simulink model "nczallcode"  (R2024a)
settings: Solver=FixedStepAuto  StartTime=0.0  StopTime=600  FixedStep=1  RelTol=1e-3
model workspace (MAT data in the model file):
  avg_loc = []
  first_column1 = []
  first_column6 = []
  locs = []
  maxValue = []
  newMaxIndex = []
  peaks = []
  stdNum = []
settings Model: Creator=LiGuoQing  LastModifiedBy=PC
settings OptimizationCC: DefaultParameterBehavior=Inlined  EnhancedBackFolding=on  PassReuseOutputArgsAs=Individual arguments  ZeroExternalMemoryAtStartup=off  ZeroInternalMemoryAtStartup=off  OptimizeBlockOrder=speed  DifferentSizesBufferReuse=on  OptimizationCustomize=off  EfficientTunableParamExpr=on
settings DebuggingCC: ParameterTunabilityLossMsg=error  UnconnectedInputMsg=warning  UnconnectedOutputMsg=warning  UnconnectedLineMsg=warning
settings HardwareCC: ProdBitPerPointer=32  ProdBitPerSizeT=32  ProdBitPerPtrDiffT=32  ProdLargestAtomicInteger=Long  ProdLargestAtomicFloat=Double  ProdWordSize=32  ProdHWDeviceType=NXP->Cortex-M4
settings ModelReferenceCC: EnableRefExpFcnMdlSchedulingChecks=on
settings SFSimCC: MATLABDynamicMemAlloc=off
settings RTWCC: Description=Embedded Coder  SystemTargetFile=ert.tlc  GenCodeOnly=on  TemplateMakefile=ert_default_tmf  GenerateReport=on  Toolchain=Microsoft Visual C++ 2019 v16.0 | nmake (64-bit Windows)  LaunchReport=on  GenerateWebview=on  GenerateCodeMetricsReport=on  GPUComputeCapability=3.5  DLArmComputeVersion=19.05
settings CodeAppCC: ForceParamTrailComments=on  IgnoreCustomStorageClasses=off  OperatorAnnotations=on  SimulinkDataObjDesc=on  SFDataObjDesc=on  InsertBlockDesc=on
settings ERTTargetCC: TargetLangStandard=C99 (ISO)  GenerateSampleERTMain=on  SupportContinuousTime=on  SupportVariableSizeSignals=on  InlinedParameterPlacement=NonHierarchical  RootIOFormat=Structure reference  ERTCustomFileTemplate=example_file_process.tlc

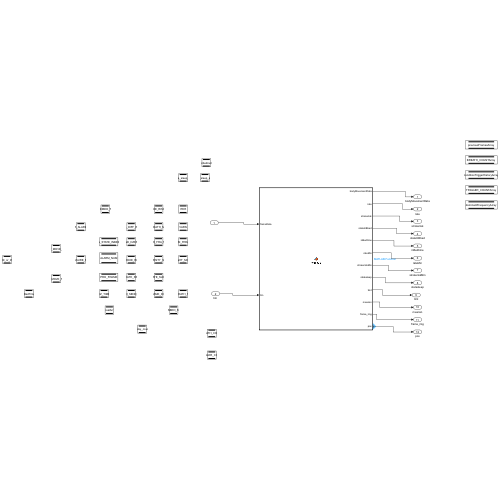
[thumbnail: Simulink's stored preview of the top-level diagram]
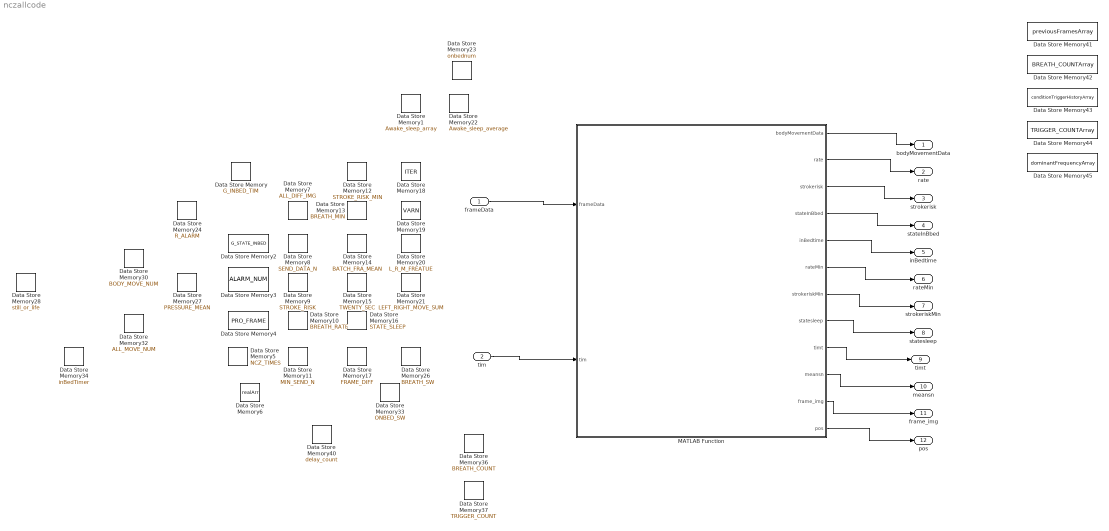
== system nczallcode ==
  frameData : Inport  OutDataTypeStr=single  PortDimensions=160
  "tim " : Inport  Port=2  OutDataTypeStr=single
  Data Store Memory : DataStoreMemory  DataStoreName=G_INBED_TIM  ReadBeforeWriteMsg=warning  WriteAfterWriteMsg=warning  WriteAfterReadMsg=warning  ShowAdditionalParam=off  OutDataTypeStr=single
  Data Store Memory1 : DataStoreMemory  DataStoreName=Awake_sleep_array  ReadBeforeWriteMsg=warning  WriteAfterWriteMsg=warning  WriteAfterReadMsg=warning  InitialValue=ones(1, 300)  ShowAdditionalParam=off  OutDataTypeStr=single
  Data Store Memory10 : DataStoreMemory  DataStoreName=BREATH_RATE  ReadBeforeWriteMsg=warning  WriteAfterWriteMsg=warning  WriteAfterReadMsg=warning  ShowAdditionalParam=off  OutDataTypeStr=single
  Data Store Memory11 : DataStoreMemory  DataStoreName=MIN_SEND_N  ReadBeforeWriteMsg=warning  WriteAfterWriteMsg=warning  WriteAfterReadMsg=warning  ShowAdditionalParam=off  OutDataTypeStr=single
  Data Store Memory12 : DataStoreMemory  DataStoreName=STROKE_RISK_MIN  ReadBeforeWriteMsg=warning  WriteAfterWriteMsg=warning  WriteAfterReadMsg=warning  ShowAdditionalParam=off  OutDataTypeStr=single
  Data Store Memory13 : DataStoreMemory  DataStoreName=BREATH_MIN  ReadBeforeWriteMsg=warning  WriteAfterWriteMsg=warning  WriteAfterReadMsg=warning  ShowAdditionalParam=off  OutDataTypeStr=single
  Data Store Memory14 : DataStoreMemory  DataStoreName=BATCH_FRA_MEAN  ReadBeforeWriteMsg=warning  WriteAfterWriteMsg=warning  WriteAfterReadMsg=warning  InitialValue=[0,0,0,0,0,0,0,0,0,0,0,0,0,0,0,0,0,0,0,0,0,0,0,0,0,0,0,0,0,0,0,0,0,0,0,0,0,0,0,0,0,0,0,0,0,0,0,0,0,0,0,0,0,0,0,0,0,0,0,0,0,0,0,0,0,0,0,0,0,0,0,0,0,0,0,0,0,0,0,0,0,0,0,0,0,0,0,0,0,0,0,0,0,0,0,0,0,0,0,0,0,0,0,0,0,0,0,0,0,0,0,0,0,0,0,0,0,0,0,0,0,0,0,0,0,0,0,0,0,0,0,0,0,0,0,0,0,0,0,0,0,0,0,0,0,0,0,0,0,0,0,0,0,0,0,0,0,0,0,0,0,0,0,0,0,0,0,0,0,0,0,0,0,0,0,0,0,0,0,0,0,0,0,0,0,0,0,0,0,0,0,0,0,0,0,0,0,0,0,0,0,0,0,0,0,0,0,0,0,0,0,0,0,0,0,0,0,0,0,0,0,0,0,0,0,0,0,0,0,0,0,0,0,0,0,0,0,0,0,0,0,0,0,0,0,0,0,0,0,0,0,0,0,0,0,0,0,0,0,0,0,0,0,0,0,0,0,0,0,0,0,0,0,0,0,0,0,0,0,0,0,0,0,0,0,0,0,0,0,0,0,0,0,0,0,0,0,0,0,0,0,0,0,0,0,0,0,0,0,0,0,0,0,0,0,0,0,0,0,0,0,0,0,0,0,0,0,0,0,0,0,0,0,0,0,0,0,0,0,0,0,0,0,0,0,0,0,0,0,0,0,0,0,0,0,0,0,0,0,0,0,0,0,0,0,0,0,0,0,0,0,0,0,0,0,0,0,0,0,0,0,0,0,0,0,0,0,0,0,0,0,0,0,0,0,0,0,0,0,0,0,0,0,0,0,0,0,0,0,0,0,0,0,0,0,0,0,0,0,0,0,0,0,0,0,0,0,0,0,0,0,0,0,0,0,0,0,0,0,0,0,0,0,0,0,0,0,0,0,0,0,0,0,0,0,0,0,0,0,0,0,0,0,0,0,0,0,0,0,0,0,0,0,0,0,0,0,0,0,0,0,0,0,0,0,0,0,0,0,0,0,0,0,0,0,0,0,0,0,0,0,0,0,0,0,0,0,0,0,0,0,0,0,0,0,0,0,0,0,0,0,0,0,0,0,0,0,0,0,0,0,0,0,0,0,0,0,0,0,0,0,0,0,0,0,0,0,0,0,0,0,0,0,0,0,0,0,0,0,0,0,0,0,0,0,0,0,0,0,0,0,0,0,0,0,0,0,0,0,0,0,0,0,0,0,0,0,0,0,0,0,0,0,0,0,0,0,0,0,0,0,0,0,0,0,0,0,0,0,0,0,0,0,0,0,0,0,0,0,0,0,0,0,0,0,0,0,0,0,0,0,0,0,0,0,0,0,0,0,0,0,0,0,0,0,0,0,0,0,0,0,0,0,0,0,0,0,0,0,0,0,0,0,0,0,0,0,0,0,0,0,0,0,0,0,0,0,0,0,0,0,0,0,0,0,0,0,0,0,0,0,0,0,0,0,0,0,0,0,0,0,0,0,0,0,0,0,0,0,0,0,0,0,0,0,0,0,0,0,0]  ShowAdditionalParam=off  OutDataTypeStr=single
  Data Store Memory15 : DataStoreMemory  DataStoreName=TWENTY_SEC  ReadBeforeWriteMsg=warning  WriteAfterWriteMsg=warning  WriteAfterReadMsg=warning  ShowAdditionalParam=off  OutDataTypeStr=single
  Data Store Memory16 : DataStoreMemory  DataStoreName=STATE_SLEEP  ReadBeforeWriteMsg=warning  WriteAfterWriteMsg=warning  WriteAfterReadMsg=warning  InitialValue=[0,0,0,0,0,0,0,0,0,0,0,0,0,0,0,0,0,0,0,0,0,0,0,0,0,0,0,0,0,0,0,0,0,0,0,0,0,0,0,0,0,0,0,0,0,0,0,0]  ShowAdditionalParam=off  OutDataTypeStr=single
  Data Store Memory17 : DataStoreMemory  DataStoreName=FRAME_DIFF  ReadBeforeWriteMsg=warning  WriteAfterWriteMsg=warning  WriteAfterReadMsg=warning  InitialValue=[0,0,0,0,0,0,0,0,0,0,0,0,0,0,0,0]  ShowAdditionalParam=off  OutDataTypeStr=single
  Data Store Memory18 : DataStoreMemory  DataStoreName=ITER  ReadBeforeWriteMsg=warning  WriteAfterWriteMsg=warning  WriteAfterReadMsg=warning  ShowAdditionalParam=off  OutDataTypeStr=single
  Data Store Memory19 : DataStoreMemory  DataStoreName=VARN  ReadBeforeWriteMsg=warning  WriteAfterWriteMsg=warning  WriteAfterReadMsg=warning  InitialValue=1  ShowAdditionalParam=off  OutDataTypeStr=single
  Data Store Memory2 : DataStoreMemory  DataStoreName=G_STATE_INBED  ReadBeforeWriteMsg=warning  WriteAfterWriteMsg=warning  WriteAfterReadMsg=warning  ShowAdditionalParam=off  OutDataTypeStr=single
  Data Store Memory20 : DataStoreMemory  DataStoreName=L_R_M_FREATUE  ReadBeforeWriteMsg=warning  WriteAfterWriteMsg=warning  WriteAfterReadMsg=warning  InitialValue=[0,0,0,0,0,0,0,0,0,0,0,0,0,0,0,0,0,0,0,0,0,0,0,0,0,0,0,0,0,0,0,0,0,0,0,0,0,0,0,0,0,0,0,0,0,0,0,0,0,0,0,0,0,0,0,0,0,0,0,0,0,0,0,0,0,0,0,0,0,0,0,0,0,0,0,0,0,0,0,0,0,0,0,0,0,0,0,0,0,0,0,0,0,0,0,0,0,0,0,0,0,0,0,0,0,0,0,0,0,0,0,0,0,0,0,0,0,0,0,0,0,0,0,0,0,0,0,0,0,0,0,0,0,0,0,0,0,0,0,0,0,0,0,0,0,0,0,0,0,0,0,0,0,0,0,0,0,0,0,0,0,0,0,0,0,0,0,0,0,0,0,0,0,0,0,0,0,0,0,0]  ShowAdditionalParam=off  OutDataTypeStr=single
  Data Store Memory21 : DataStoreMemory  DataStoreName=LEFT_RIGHT_MOVE_SUM  ReadBeforeWriteMsg=warning  WriteAfterWriteMsg=warning  WriteAfterReadMsg=warning  InitialValue=[0,0,0,0]  ShowAdditionalParam=off  OutDataTypeStr=single
  Data Store Memory22 : DataStoreMemory  DataStoreName=Awake_sleep_average  ReadBeforeWriteMsg=warning  WriteAfterWriteMsg=warning  WriteAfterReadMsg=warning  InitialValue=zeros(1,48)  ShowAdditionalParam=off  OutDataTypeStr=double
  Data Store Memory23 : DataStoreMemory  DataStoreName=onbednum  ReadBeforeWriteMsg=warning  WriteAfterWriteMsg=warning  WriteAfterReadMsg=warning  ShowAdditionalParam=off  OutDataTypeStr=double
  Data Store Memory24 : DataStoreMemory  DataStoreName=R_ALARM  ReadBeforeWriteMsg=warning  WriteAfterWriteMsg=warning  WriteAfterReadMsg=warning  InitialValue=[0,0,0,0,0,0,0,0,0,0,0,0,0,0,0,0,0,0,0,0,0,0,0,0,0,0,0,0,0,0,0,0,0,0,0,0,0,0,0,0,0,0,0,0,0,0,0,0,0,0,0,0,0,0,0,0,0,0,0,0,0,0,0,0,0,0,0,0,0,0,0,0,0,0,0,0,0,0,0,0,0,0,0,0,0,0,0,0,0,0,0,0,0,0,0,0,0,0,0,0,0,0,0,0,0,0,0,0,0,0,0,0,0,0,0,0,0,0,0,0,0,0,0,0,0,0,0,0,0,0,0,0,0,0,0,0,0,0,0,0,0,0,0,0,0,0,0,0,0,0,0,0,0,0,0,0,0,0,0,0,0,0,0,0,0,0,0,0,0,0,0,0,0,0,0,0,0,0,0,0]  ShowAdditionalParam=off  OutDataTypeStr=single
  Data Store Memory26 : DataStoreMemory  DataStoreName=BREATH_SW  ReadBeforeWriteMsg=warning  WriteAfterWriteMsg=warning  WriteAfterReadMsg=warning  ShowAdditionalParam=off  OutDataTypeStr=single
  Data Store Memory27 : DataStoreMemory  DataStoreName=PRESSURE_MEAN  ReadBeforeWriteMsg=warning  WriteAfterWriteMsg=warning  WriteAfterReadMsg=warning  ShowAdditionalParam=off  OutDataTypeStr=single
  Data Store Memory28 : DataStoreMemory  DataStoreName=still_or_life  ReadBeforeWriteMsg=warning  WriteAfterWriteMsg=warning  WriteAfterReadMsg=warning  ShowAdditionalParam=off  OutDataTypeStr=single
  Data Store Memory3 : DataStoreMemory  DataStoreName=ALARM_NUM  ReadBeforeWriteMsg=warning  WriteAfterWriteMsg=warning  WriteAfterReadMsg=warning  ShowAdditionalParam=off  OutDataTypeStr=single
  Data Store Memory30 : DataStoreMemory  DataStoreName=BODY_MOVE_NUM  ReadBeforeWriteMsg=warning  WriteAfterWriteMsg=warning  WriteAfterReadMsg=warning  ShowAdditionalParam=off  OutDataTypeStr=single
  Data Store Memory32 : DataStoreMemory  DataStoreName=ALL_MOVE_NUM  ReadBeforeWriteMsg=warning  WriteAfterWriteMsg=warning  WriteAfterReadMsg=warning  ShowAdditionalParam=off  OutDataTypeStr=single
  Data Store Memory33 : DataStoreMemory  DataStoreName=ONBED_SW  ReadBeforeWriteMsg=warning  WriteAfterWriteMsg=warning  WriteAfterReadMsg=warning  ShowAdditionalParam=off  OutDataTypeStr=single
  Data Store Memory34 : DataStoreMemory  DataStoreName=inBedTimer  ReadBeforeWriteMsg=warning  WriteAfterWriteMsg=warning  WriteAfterReadMsg=warning  ShowAdditionalParam=off  OutDataTypeStr=single
  Data Store Memory36 : DataStoreMemory  DataStoreName=BREATH_COUNT  ReadBeforeWriteMsg=warning  WriteAfterWriteMsg=warning  WriteAfterReadMsg=warning  ShowAdditionalParam=off  OutDataTypeStr=double
  Data Store Memory37 : DataStoreMemory  DataStoreName=TRIGGER_COUNT  ReadBeforeWriteMsg=warning  WriteAfterWriteMsg=warning  WriteAfterReadMsg=warning  ShowAdditionalParam=off  OutDataTypeStr=double
  Data Store Memory4 : DataStoreMemory  DataStoreName=PRO_FRAME  ReadBeforeWriteMsg=warning  WriteAfterWriteMsg=warning  WriteAfterReadMsg=warning  InitialValue=[0,0,0,0,0,0,0,0,0,0,0,0,0,0,0,0;0,0,0,0,0,0,0,0,0,0,0,0,0,0,0,0;0,0,0,0,0,0,0,0,0,0,0,0,0,0,0,0;0,0,0,0,0,0,0,0,0,0,0,0,0,0,0,0;0,0,0,0,0,0,0,0,0,0,0,0,0,0,0,0;0,0,0,0,0,0,0,0,0,0,0,0,0,0,0,0;0,0,0,0,0,0,0,0,0,0,0,0,0,0,0,0;0,0,0,0,0,0,0,0,0,0,0,0,0,0,0,0;0,0,0,0,0,0,0,0,0,0,0,0,0,0,0,0;0,0,0,0,0,0,0,0,0,0,0,0,0,0,0,0]  ShowAdditionalParam=off  OutDataTypeStr=single
  Data Store Memory40 : DataStoreMemory  DataStoreName=delay_count  ReadBeforeWriteMsg=warning  WriteAfterWriteMsg=warning  WriteAfterReadMsg=warning  InitialValue=20  ShowAdditionalParam=off  OutDataTypeStr=double
  Data Store Memory41 : DataStoreMemory  DataStoreName=previousFramesArray  ReadBeforeWriteMsg=warning  WriteAfterWriteMsg=warning  WriteAfterReadMsg=warning  InitialValue=zeros(96,16)  ShowAdditionalParam=off  OutDataTypeStr=double
  Data Store Memory42 : DataStoreMemory  DataStoreName=BREATH_COUNTArray  ReadBeforeWriteMsg=warning  WriteAfterWriteMsg=warning  WriteAfterReadMsg=warning  InitialValue=zeros(1, 16)  ShowAdditionalParam=off  OutDataTypeStr=double
  Data Store Memory43 : DataStoreMemory  DataStoreName=conditionTriggerHistoryArray  ReadBeforeWriteMsg=warning  WriteAfterWriteMsg=warning  WriteAfterReadMsg=warning  InitialValue=false(5,16)  ShowAdditionalParam=off  OutDataTypeStr=double
  Data Store Memory44 : DataStoreMemory  DataStoreName=TRIGGER_COUNTArray  ReadBeforeWriteMsg=warning  WriteAfterWriteMsg=warning  WriteAfterReadMsg=warning  InitialValue=zeros(1,16)  ShowAdditionalParam=off  OutDataTypeStr=double
  Data Store Memory45 : DataStoreMemory  DataStoreName=dominantFrequencyArray  ReadBeforeWriteMsg=warning  WriteAfterWriteMsg=warning  WriteAfterReadMsg=warning  InitialValue=zeros(1,16)  ShowAdditionalParam=off  OutDataTypeStr=double
  Data Store Memory5 : DataStoreMemory  DataStoreName=NCZ_TIMES  ReadBeforeWriteMsg=warning  WriteAfterWriteMsg=warning  WriteAfterReadMsg=warning  ShowAdditionalParam=off  OutDataTypeStr=single
  Data Store Memory6 : DataStoreMemory  DataStoreName=realArr  ReadBeforeWriteMsg=warning  WriteAfterWriteMsg=warning  WriteAfterReadMsg=warning  InitialValue=zeros(100, 40)  ShowAdditionalParam=off  OutDataTypeStr=single
  Data Store Memory7 : DataStoreMemory  DataStoreName=ALL_DIFF_IMG  ReadBeforeWriteMsg=warning  WriteAfterWriteMsg=warning  WriteAfterReadMsg=warning  InitialValue=[0,0,0,0,0,0,0,0,0,0,0,0,0,0,0,0,0,0,0,0,0,0,0,0]  ShowAdditionalParam=off  OutDataTypeStr=single
  Data Store Memory8 : DataStoreMemory  DataStoreName=SEND_DATA_N  ReadBeforeWriteMsg=warning  WriteAfterWriteMsg=warning  WriteAfterReadMsg=warning  ShowAdditionalParam=off  OutDataTypeStr=single
  Data Store Memory9 : DataStoreMemory  DataStoreName=STROKE_RISK  ReadBeforeWriteMsg=warning  WriteAfterWriteMsg=warning  WriteAfterReadMsg=warning  ShowAdditionalParam=off  OutDataTypeStr=single
  MATLAB Function : MATLAB Function  TreatAsAtomicUnit=on
  bodyMovementData : Outport  OutDataTypeStr=single
  rate : Outport  Port=2  OutDataTypeStr=single
  strokerisk : Outport  Port=3  OutDataTypeStr=single
  stateInBbed : Outport  Port=4  OutDataTypeStr=single
  inBedtime : Outport  Port=5  OutDataTypeStr=single
  rateMin : Outport  Port=6  OutDataTypeStr=single
  strokeriskMin : Outport  Port=7  OutDataTypeStr=single
  statesleep : Outport  Port=8  OutDataTypeStr=single
  timt : Outport  Port=9  OutDataTypeStr=single
  meansn : Outport  Port=10  OutDataTypeStr=single
  frame_img : Outport  Port=11  OutDataTypeStr=single
  pos : Outport  Port=12  OutDataTypeStr=single
  wires:
  frameData/1 -> MATLAB Function/1(frameData)
  MATLAB Function/1(bodyMovementData) -> bodyMovementData/1
  MATLAB Function/2(rate) -> rate/1
  MATLAB Function/3(strokerisk) -> strokerisk/1
  MATLAB Function/4(stateInBbed) -> stateInBbed/1
  MATLAB Function/5(inBedtime) -> inBedtime/1
  MATLAB Function/6(rateMin) -> rateMin/1
  MATLAB Function/7(strokeriskMin) -> strokeriskMin/1
  MATLAB Function/8(statesleep) -> statesleep/1
  MATLAB Function/9(timt) -> timt/1
  MATLAB Function/10(meansn) -> meansn/1
  "tim "/1 -> MATLAB Function/2(tim)
  MATLAB Function/11(frame_img) -> frame_img/1
  MATLAB Function/12(pos) -> pos/1

== matlab function nczallcode/MATLAB Function ==
  data: bodyMovementData output; rate output; strokerisk output; stateInBbed output; inBedtime output; rateMin output; strokeriskMin output; statesleep output; frameData input; G_INBED_TIM data_store_memory; G_STATE_INBED data_store_memory; PRO_FRAME data_store_memory; NCZ_TIMES data_store_memory; ALL_DIFF_IMG data_store_memory; SEND_DATA_N data_store_memory; STROKE_RISK data_store_memory; BREATH_RATE data_store_memory; MIN_SEND_N data_store_memory; STROKE_RISK_MIN data_store_memory; BREATH_MIN data_store_memory; BATCH_FRA_MEAN data_store_memory; TWENTY_SEC data_store_memory; STATE_SLEEP data_store_memory; FRAME_DIFF data_store_memory; ITER data_store_memory; timt output; VARN data_store_memory; meansn output; tim input; BREATH_SW data_store_memory; PRESSURE_MEAN data_store_memory; L_R_M_FREATUE data_store_memory; LEFT_RIGHT_MOVE_SUM data_store_memory; R_ALARM data_store_memory; ALARM_NUM data_store_memory; BODY_MOVE_NUM data_store_memory; ALL_MOVE_NUM data_store_memory; still_or_life data_store_memory; frame_img output; realArr data_store_memory; ONBED_SW data_store_memory; inBedTimer data_store_memory; BREATH_COUNT data_store_memory; TRIGGER_COUNT data_store_memory; delay_count data_store_memory; previousFramesArray data_store_memory; BREATH_COUNTArray data_store_memory; conditionTriggerHistoryArray data_store_memory; TRIGGER_COUNTArray data_store_memory; dominantFrequencyArray data_store_memory; Awake_sleep_array data_store_memory; Awake_sleep_average data_store_memory; onbednum data_store_memory; pos output
function [bodyMovementData,rate,strokerisk,stateInBbed,inBedtime,rateMin,strokeriskMin,statesleep,timt,meansn,frame_img, pos] = nczcode(frameData, tim)
    % 定义全局变量
    global G_INBED_TIM 
%     global G_OUTBED_TIM
%     global SW_INBED
%     global SW_OUTBED
%     global INBED_TIME %Bed leaving reminder record variable
    global realArr
%     global onBedArr
    global G_STATE_INBED
    global PRO_FRAME
    global ALL_DIFF_IMG
    global SEND_DATA_N  
    global STROKE_RISK
    global BREATH_RATE  
    global MIN_SEND_N
    global STROKE_RISK_MIN
    global BREATH_MIN
    global BATCH_FRA_MEAN
    global TWENTY_SEC       
    global STATE_SLEEP
    global FRAME_DIFF
    global ITER
    global VARN
%     global ONBED_SW
    global BREATH_SW
    global PRESSURE_MEAN
    global BODY_MOVE_NUM
%     global ALL_MOVE_LIST
%     global ALL_MOVE_NUM
    global still_or_life
    global inBedTimer
%     global previousFrames
%     global BREATH_COUNT
%     global TRIGGER_COUNT
%     global conditionTriggerHistory %still state trigger
%     global dominantFrequency
    global delay_count
    %清醒入睡数组
    global Awake_sleep_array
    global Awake_sleep_average
    %onbednum 在床持续时间计数
    global onbednum
      
      div_num = 6; %160大床整除系数
      XTest = frameData';
      frameData = round(frameData/div_num);
    % 调整数据顺序并去噪
    frameData_b = frameData; % copy of original data for breath

    framedata_fall = frameData_b';
   

    %% 初始化相关变量
    inBedFlag = 14 * VARN; %0621：2000/160
%     move_prop = VARN;
    bodyMovementData = (-1) * ones(24,1) * VARN;   
    strokerisk = (-1) * VARN;  
    strokeriskMin = (-1) * VARN;   
    rate = (-1) * VARN;
    rateMin = (-1) * VARN;
    stateInBbed = (-1) * VARN;    
    statesleep = (-1) * ones(48,1) * VARN; 
    inBedtime = (-1) * VARN;
    timt = (-1) * VARN;
    meansn = (-1) * VARN;
    pos = (-1) * VARN;
    frame_img = (-1) * ones(160,1) * VARN;
%     samplingRate = 12 * VARN;
%     alarm_switch = 0;
%     on_mat_flag = 0; %在垫标志位240703
    SEND_DATA_N = SEND_DATA_N+1;

    %% 体动赋值
    gain = 1;
    if SEND_DATA_N*gain >= 4  
        pos = single(predictTree(XTest));
%         rate = BODY_MOVE_NUM;%测试
        BREATH_MIN = BREATH_MIN + BREATH_RATE;
        SEND_DATA_N = VARN - 1;
        still_or_life = VARN - 1;
    end

    %% 数据处理和传输
    if MIN_SEND_N*gain >= 720
        frame_img = reshape(frameData, 160, 1);
    end
end

%% 辅助函数

function YPred = predictTree(XTest)
    % 加载预训练的决策树模型
    persistent treeModel
    if isempty(treeModel)
        treeModel = loadCompactModel('trainedTreeModel.mat');
    end
    
    % 对输入数据进行归一化
    X_min = min(XTest, [], 2);
    X_max = max(XTest, [], 2);
    XTest_normalized = (XTest - X_min) ./ (X_max - X_min + eps);
    
    % 预测
    YPred = predict(treeModel, XTest_normalized);
end

function model = loadCompactModel(filename)
    % 加载紧凑模型
    s = coder.load(filename);
    model = s.tree;  % 将 s.treeModel 改为 s.tree
end
